simulink model "EMG_FES2(backup-18-05-2018)"  (R2014a)
settings: Solver=FixedStepDiscrete  StartTime=0.0  StopTime=inf  FixedStep=1/aFES.Fs  RelTol=1e-3
InitFcn:
  | mdl_initFcn_
StopFcn:
  | mdl_stopFcn_
values from neighbouring files (symbols this model uses):
  aFES = emgfes_feedback(aFES,[0,0,0,round(rand(1,2)*100)],1)    [emgfes_feedback_simulation.m]    (also in emgfesgui.m = a.aFES)
undefined symbols (not defined in the file or in its folder): analoginput, emgfes_feedback
libraries: dspmtrx3 x4, dspswit3 x3, simulink x2, ScienceStimHasomed_Lib x2, dspinverses x2, daqlib x1
settings Model: Creator=bethel.osuagwu  LastModifiedBy=bethel.osuagwu

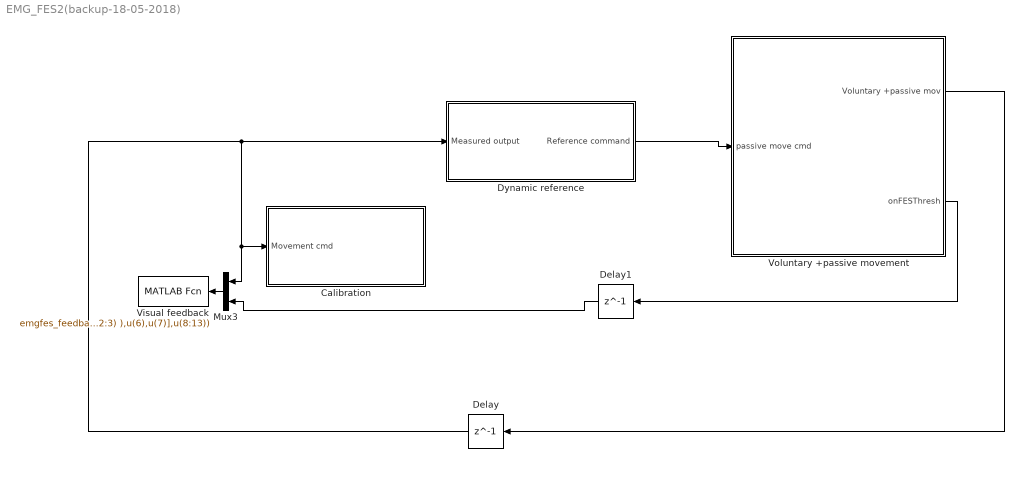
== system EMG_FES2(backup-18-05-2018) ==
  Calibration : Subsystem
  Delay : Delay  DelayLength=1  InitialCondition=zeros(7,1)
  Delay1 : Delay  DelayLength=1  InitialCondition=zeros(6,1)
  Dynamic reference : Subsystem
  Mux3 : Mux  Inputs=2
  Visual feedback : MATLABFcn  MATLABFcn=emgfes_feedback(aFES,[u(1), (u(2:3)'-aFES.activeSensorMin(2:3))./(aFES.activeSensorMax(2:3)-aFES.activeSensorMin(2:3) ),u(6),u(7)],u(8:13))  OutputDimensions=0
  Voluntary +passive movement : Subsystem
  wires:
  Dynamic reference/1(Reference command) -> Voluntary +passive movement/1(passive move cmd)
  Voluntary +passive movement/1(Voluntary +passive mov) -> Delay/1
  Delay/1 -> Dynamic reference/1(Measured output), Calibration/1(Movement cmd), Mux3/1
  Voluntary +passive movement/2(onFESThresh) -> Delay1/1
  Mux3/1 -> Visual feedback/1
  Delay1/1 -> Mux3/2

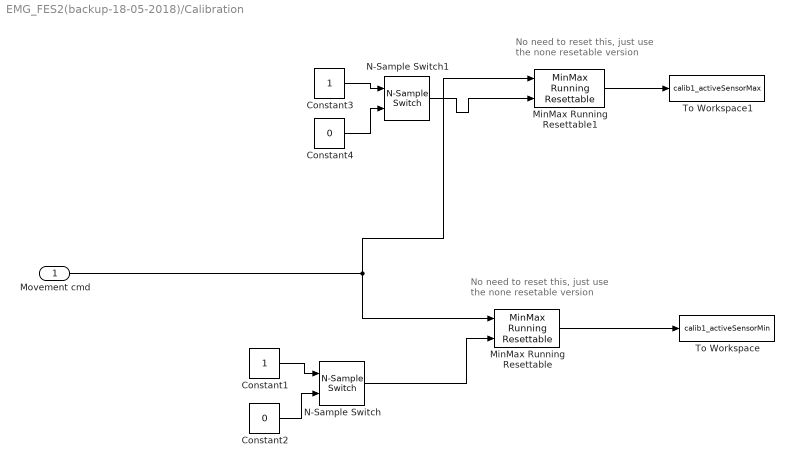
== system EMG_FES2(backup-18-05-2018)/Calibration ==
  note: No need to reset this, just use
      |  the none resetable version
  note: No need to reset this, just use
      |  the none resetable version
  Movement cmd : Inport
  Constant1 : Constant
  Constant2 : Constant  Value=0
  Constant3 : Constant
  Constant4 : Constant  Value=0
  MinMax Running Resettable : simulink/Math Operations/MinMax Running Resettable  Function=min  vinit=inf
  MinMax Running Resettable1 : simulink/Math Operations/MinMax Running Resettable  Function=max  vinit=-inf
  N-Sample Switch : dspswit3/N-Sample Switch  N=10000  reset=off  TriggerType=Rising edge  Ts=-1
  N-Sample Switch1 : dspswit3/N-Sample Switch  N=10000  reset=off  TriggerType=Rising edge  Ts=-1
  To Workspace : ToWorkspace  VariableName=calib1_activeSensorMin  SampleTime=-1
      settings: MaxDataPoints=1
  To Workspace1 : ToWorkspace  VariableName=calib1_activeSensorMax  SampleTime=-1
      settings: MaxDataPoints=1
  wires:
  N-Sample Switch1/1 -> MinMax Running Resettable1/2
  Constant1/1 -> N-Sample Switch/1
  MinMax Running Resettable1/1 -> To Workspace1/1
  MinMax Running Resettable/1 -> To Workspace/1
  N-Sample Switch/1 -> MinMax Running Resettable/2
  Constant2/1 -> N-Sample Switch/2
  Constant3/1 -> N-Sample Switch1/1
  Constant4/1 -> N-Sample Switch1/2
  Movement cmd/1 -> MinMax Running Resettable1/1, MinMax Running Resettable/1

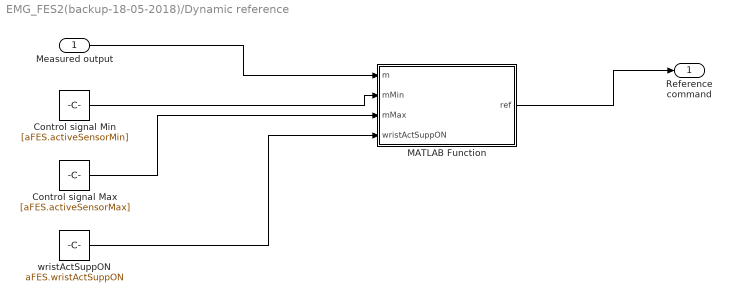
== system EMG_FES2(backup-18-05-2018)/Dynamic reference ==
  Measured output : Inport
  Control signal Max : Constant  Value=[aFES.activeSensorMax]
  Control signal Min : Constant  Value=[aFES.activeSensorMin]
  MATLAB Function : MATLAB Function  TreatAsAtomicUnit=on
  wristActSuppON : Constant  Value=aFES.wristActSuppON
  Reference command : Outport
  wires:
  Measured output/1 -> MATLAB Function/1(m)
  MATLAB Function/1(ref) -> Reference command/1
  Control signal Min/1 -> MATLAB Function/2(mMin)
  Control signal Max/1 -> MATLAB Function/3(mMax)
  wristActSuppON/1 -> MATLAB Function/4(wristActSuppON)

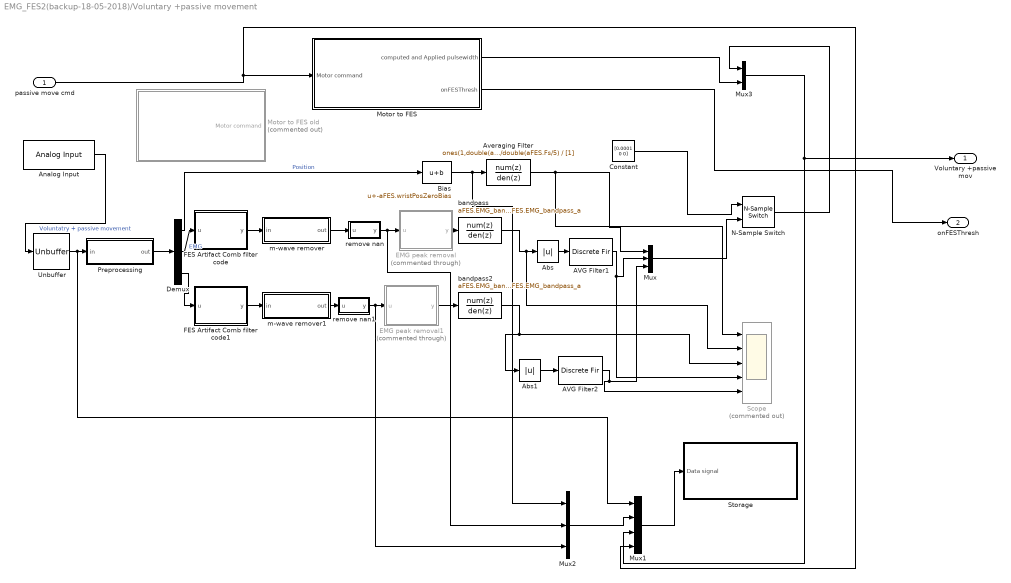
== system EMG_FES2(backup-18-05-2018)/Voluntary +passive movement ==
  passive move cmd : Inport
  " AVG Filter1" : DiscreteFir  Coefficients=ones(1,1000)/1000
  " AVG Filter2" : DiscreteFir  Coefficients=ones(1,1000)/1000
  Abs : Abs
  Abs1 : Abs
  Analog Input : daqlib/Analog Input  AcqMode=0  DeviceMenu=nidaq Dev1 (USB-6341 (BNC))  Device=nidaq Dev1 (USB-6341 (BNC))  ObjConstructor=analoginput('nidaq','Dev1')  SampleRate=1000  ActualRate=1000  SamplesPerFrame=2  InputType=Differential  NChannelsSelected=3  Channels=1$0$$2$#1$1$$2$#1$2$$2$#0$3$$1$#0$4$$1$#0$5$$1$#0$6$$1$#0$7$$1$#  NPorts=1 for all hardware channels  DataType=double
      settings: SignalType=Sample-based
  Averaging Filter : DiscreteFilter  Numerator=ones(1,double(aFES.Fs/5))/double(aFES.Fs/5)  Denominator=[1]
  Bias : Bias  Bias=-aFES.wristPosZeroBias
  Constant : Constant  Value=[0.0001 0 0]
  Demux : Demux  Outputs=3
  EMG peak removal : MATLAB Function  Commented=through  TreatAsAtomicUnit=on
  EMG peak removal1 : MATLAB Function  Commented=through  TreatAsAtomicUnit=on
  FES Artifact Comb filter code : MATLAB Function  TreatAsAtomicUnit=on
  FES Artifact Comb filter code1 : MATLAB Function  TreatAsAtomicUnit=on
  Motor to FES : Subsystem
  Motor to FES old : Subsystem  Commented=on
  Mux : Mux  Inputs=3
  Mux1 : Mux
  Mux2 : Mux  Inputs=3
  Mux3 : Mux  Inputs=2
  N-Sample Switch : dspswit3/N-Sample Switch  N=10  reset=off  TriggerType=Rising edge  Ts=-1
  Preprocessing : Subsystem
  Scope : Scope  Commented=on  NumInputPorts=5
      settings: YMin=-0.45~-0.15~-0.15~0~0  YMax=2.77556e-17~0.2~0.125~0.0125~0.015
  Storage : Subsystem
  Unbuffer : Unbuffer  SampleBasedProcessing=Same as frame based
  bandpass : DiscreteFilter  Numerator=aFES.EMG_bandpass_b  Denominator=aFES.EMG_bandpass_a
  bandpass2 : DiscreteFilter  Numerator=aFES.EMG_bandpass_b  Denominator=aFES.EMG_bandpass_a
  m-wave remover : Subsystem
  m-wave remover1 : Subsystem
  remove nan : MATLAB Function  TreatAsAtomicUnit=on
  remove nan1 : MATLAB Function  TreatAsAtomicUnit=on
  Voluntary +passive mov : Outport
  onFESThresh : Outport  Port=2
  wires:
  Analog Input/1 -> Unbuffer/1  "Voluntatry + passive movement"
  Demux/1 -> Bias/1  "Position"
  Abs/1 -> " AVG Filter1"/1
  " AVG Filter1"/1 -> Scope/4, Mux/2
  passive move cmd/1 -> Mux1/4, Motor to FES/1(Motor command)
  Demux/2 -> FES Artifact Comb filter code/1(u)  "EMG"
  Constant/1 -> N-Sample Switch/1
  N-Sample Switch/1 -> Mux3/1
  Unbuffer/1 -> Mux1/1, Preprocessing/1(in)
  Bias/1 -> Mux2/1, Averaging Filter/1
  Averaging Filter/1 -> Scope/1, Mux/1
  Abs1/1 -> " AVG Filter2"/1
  " AVG Filter2"/1 -> Scope/5, Mux/3
  Demux/3 -> FES Artifact Comb filter code1/1(u)
  FES Artifact Comb filter code/1(y) -> m-wave remover/1(in)
  EMG peak removal1/1(y) -> bandpass2/1
  Mux/1 -> N-Sample Switch/2
  Preprocessing/1(out) -> Demux/1
  m-wave remover/1(out) -> remove nan/1(u)
  FES Artifact Comb filter code1/1(y) -> m-wave remover1/1(in)
  EMG peak removal/1(y) -> bandpass/1
  bandpass/1 -> Scope/2, Abs/1
  bandpass2/1 -> Abs1/1, Scope/3
  remove nan/1(y) -> Mux2/2, EMG peak removal/1(u)
  remove nan1/1(y) -> Mux2/3, EMG peak removal1/1(u)
  m-wave remover1/1(out) -> remove nan1/1(u)
  Mux1/1 -> Storage/1(Data signal)
  Mux2/1 -> Mux1/2
  Motor to FES/1(computed and Applied pulsewidth) -> Mux3/2
  Motor to FES/2(onFESThresh) -> onFESThresh/1
  Mux3/1 -> Voluntary +passive mov/1, Mux1/3

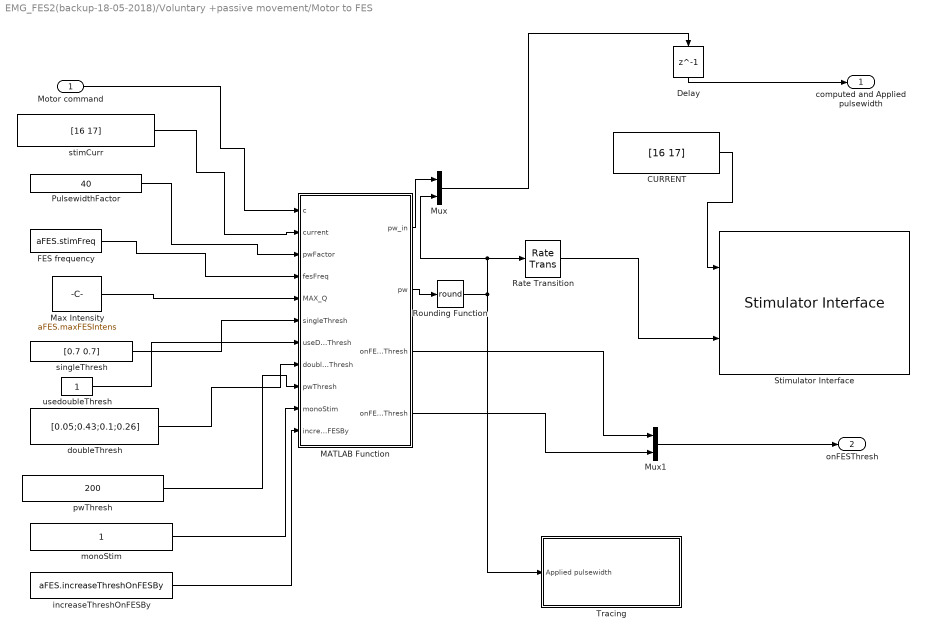
== system EMG_FES2(backup-18-05-2018)/Voluntary +passive movement/Motor to FES ==
  Motor command : Inport
  CURRENT : Constant  Value=[16 17]
  Delay : Delay  DelayLength=1  InitialCondition=0
  FES frequency : Constant  Value=aFES.stimFreq
  MATLAB Function : MATLAB Function  TreatAsAtomicUnit=on
  Max Intensity : Constant  Value=aFES.maxFESIntens
  Mux : Mux  Inputs=2
  Mux1 : Mux  Inputs=2
  PulsewidthFactor : Constant  Value=40
  Rate Transition : RateTransition
  Rounding Function : Rounding  Operator=round
  Stimulator Interface : ScienceStimHasomed_Lib/Stimulator Interface  Ts=33/aFES.Fs  com_port=COM9  channelstim=[1,2]  tsone=round((1/aFES.stimFreq)*1000)  tstwo=5  channellf=[]  nfactor=[]  outflag=off  dtflag=off
  Tracing : Subsystem
  doubleThresh : Constant  Value=[0.05;0.43;0.1;0.26]
  increaseThreshOnFESBy : Constant  Value=aFES.increaseThreshOnFESBy
  monoStim : Constant
  pwThresh : Constant  Value=200
  singleThresh : Constant  Value=[0.7 0.7]
  stimCurr : Constant  Value=[16 17]
  usedoubleThresh : Constant
  computed and Applied pulsewidth : Outport
  onFESThresh : Outport  Port=2
  wires:
  CURRENT/1 -> Stimulator Interface/1
  Motor command/1 -> MATLAB Function/1(c)
  MATLAB Function/2(pw) -> Rounding Function/1
  Rate Transition/1 -> Stimulator Interface/2
  stimCurr/1 -> MATLAB Function/2(current)
  Max Intensity/1 -> MATLAB Function/5(MAX_Q)
  doubleThresh/1 -> MATLAB Function/8(doubleThresh)
  MATLAB Function/1(pw_in) -> Mux/1
  Rounding Function/1 -> Tracing/1(Applied pulsewidth), Mux/2, Rate Transition/1
  pwThresh/1 -> MATLAB Function/9(pwThresh)
  FES frequency/1 -> MATLAB Function/4(fesFreq)
  PulsewidthFactor/1 -> MATLAB Function/3(pwFactor)
  monoStim/1 -> MATLAB Function/10(monoStim)
  Delay/1 -> computed and Applied pulsewidth/1
  usedoubleThresh/1 -> MATLAB Function/7(useDoubleThresh)
  singleThresh/1 -> MATLAB Function/6(singleThresh)
  Mux/1 -> Delay/1
  increaseThreshOnFESBy/1 -> MATLAB Function/11(increaseThreshOnFESBy)
  MATLAB Function/3(onFESSingleThresh) -> Mux1/1
  MATLAB Function/4(onFESDoubleThresh) -> Mux1/2
  Mux1/1 -> onFESThresh/1

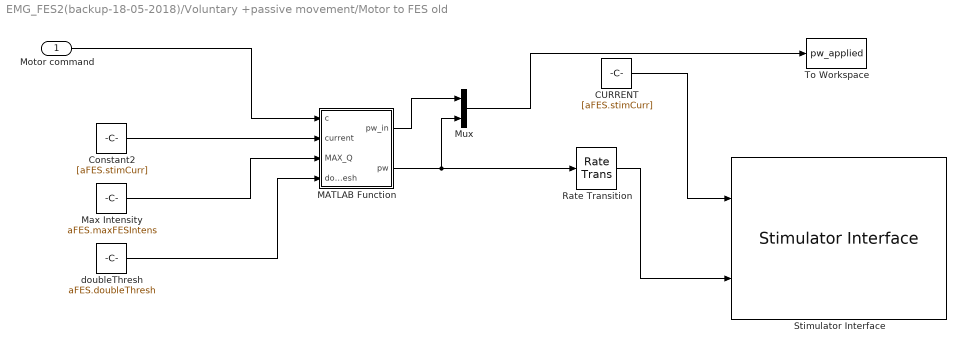
== system EMG_FES2(backup-18-05-2018)/Voluntary +passive movement/Motor to FES old ==
  Motor command : Inport
  CURRENT : Constant  Value=[aFES.stimCurr]
  Constant2 : Constant  Value=[aFES.stimCurr]
  MATLAB Function : MATLAB Function  TreatAsAtomicUnit=on
  Max Intensity : Constant  Value=aFES.maxFESIntens
  Mux : Mux  Inputs=2
  Rate Transition : RateTransition
  Stimulator Interface : ScienceStimHasomed_Lib/Stimulator Interface  Ts=33/aFES.Fs  com_port=COM9  channelstim=[1,2]  tsone=round((1/aFES.stimFreq)*1000)  tstwo=5  channellf=[]  nfactor=[]  outflag=off  dtflag=off
  To Workspace : ToWorkspace  VariableName=pw_applied  SampleTime=-1
  doubleThresh : Constant  Value=aFES.doubleThresh
  wires:
  Mux/1 -> To Workspace/1
  MATLAB Function/1(pw_in) -> Mux/1
  doubleThresh/1 -> MATLAB Function/4(doubleThresh)
  Max Intensity/1 -> MATLAB Function/3(MAX_Q)
  Constant2/1 -> MATLAB Function/2(current)
  Rate Transition/1 -> Stimulator Interface/2
  MATLAB Function/2(pw) -> Rate Transition/1, Mux/2
  Motor command/1 -> MATLAB Function/1(c)
  CURRENT/1 -> Stimulator Interface/1

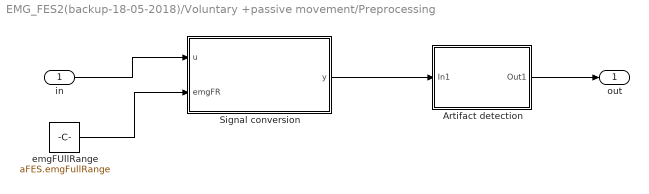
== system EMG_FES2(backup-18-05-2018)/Voluntary +passive movement/Preprocessing ==
  in : Inport
  Artifact detection : Subsystem
  Signal conversion : MATLAB Function  TreatAsAtomicUnit=on
  emgFUllRange : Constant  Value=aFES.emgFullRange
  out : Outport
  wires:
  Signal conversion/1(y) -> Artifact detection/1(In1)
  in/1 -> Signal conversion/1(u)
  Artifact detection/1(Out1) -> out/1
  emgFUllRange/1 -> Signal conversion/2(emgFR)

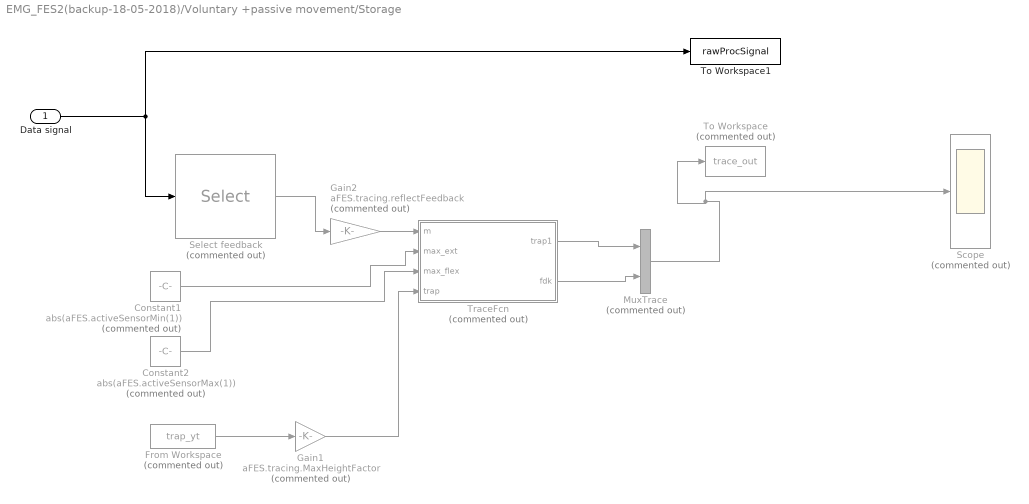
== system EMG_FES2(backup-18-05-2018)/Voluntary +passive movement/Storage ==
  Data signal : Inport
  Constant1 : Constant  Commented=on  Value=abs(aFES.activeSensorMin(1))
  Constant2 : Constant  Commented=on  Value=abs(aFES.activeSensorMax(1))
  From Workspace : FromWorkspace  Commented=on  VariableName=trap_yt  SampleTime=1/aFES.Fs  OutputAfterFinalValue=Setting to zero
  Gain1 : Gain  Commented=on  Gain=aFES.tracing.MaxHeightFactor
  Gain2 : Gain  Commented=on  Gain=aFES.tracing.reflectFeedback
  MuxTrace : Mux  Commented=on  Inputs=2
  Scope : Scope  Commented=on
      settings: TimeRange=100  YMin=-2.25  YMax=2  SaveName=ScopeData2
  Select feedback : Selector  Commented=on  InputPortWidth=9  Indices=[7]
  To Workspace : ToWorkspace  Commented=on  VariableName=trace_out  SampleTime=-1
  To Workspace1 : ToWorkspace  VariableName=rawProcSignal  SampleTime=-1
  TraceFcn : MATLAB Function  Commented=on  TreatAsAtomicUnit=on
  wires:
  TraceFcn/1(trap1) -> MuxTrace/1
  MuxTrace/1 -> Scope/1, To Workspace/1
  Gain1/1 -> TraceFcn/4(trap)
  Constant1/1 -> TraceFcn/2(max_ext)
  Constant2/1 -> TraceFcn/3(max_flex)
  Data signal/1 -> Select feedback/1, To Workspace1/1
  From Workspace/1 -> Gain1/1
  TraceFcn/2(fdk) -> MuxTrace/2
  Select feedback/1 -> Gain2/1
  Gain2/1 -> TraceFcn/1(m)

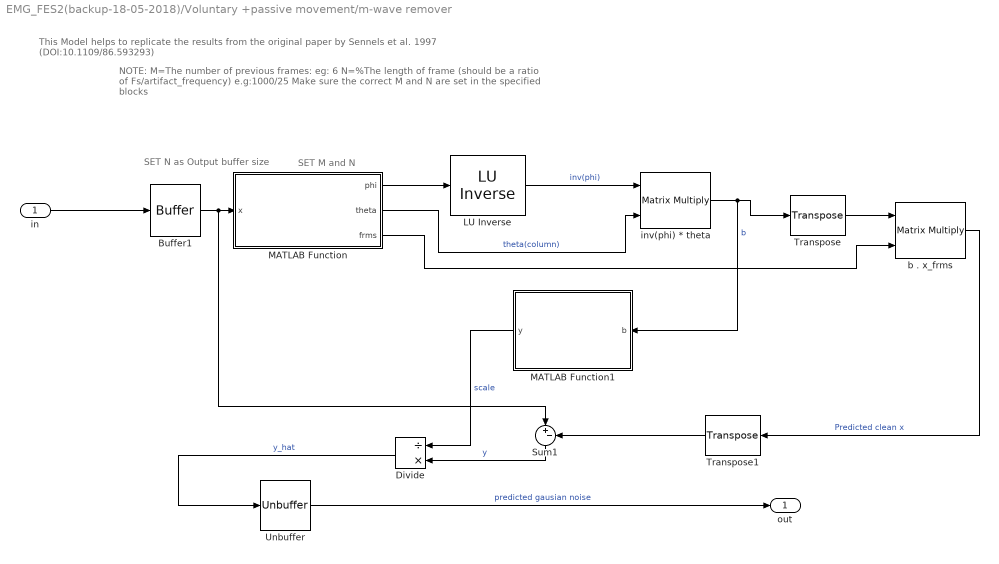
== system EMG_FES2(backup-18-05-2018)/Voluntary +passive movement/m-wave remover ==
  note: NOTE:
      | M=The number of previous frames: eg: 6
      | N=%The length of frame (should be a ratio of Fs/artifact_frequency) e.g:1000/25
      | Make sure the correct M and N are set in the specified blocks
  note: SET N as Output
      | buffer size
  note: SET M and N
  note: This Model helps to replicate the results from the original paper by Sennels et al. 1997 (DOI:10.1109/86.593293)
  in : Inport
  " LU Inverse" : dspinverses/ LU Inverse
  Buffer1 : Buffer  N=40  TreatMby1Signals=One channel
  Divide : Product  Inputs=/*
  MATLAB Function : MATLAB Function  TreatAsAtomicUnit=on
  MATLAB Function1 : MATLAB Function  TreatAsAtomicUnit=on
  Sum1 : Sum  Inputs=|+-
  Transpose : dspmtrx3/Transpose  Hermitian=off  overflowFlag=off
  Transpose1 : dspmtrx3/Transpose  Hermitian=off  overflowFlag=off
  Unbuffer : Unbuffer  SampleBasedProcessing=Same as frame based
  b . x_frms : Product  Multiplication=Matrix(*)
  inv(phi) * theta : Product  Multiplication=Matrix(*)
  out : Outport
  wires:
  Buffer1/1 -> Sum1/1, MATLAB Function/1(x)
  MATLAB Function/1(phi) -> " LU Inverse"/1
  MATLAB Function/2(theta) -> inv(phi) * theta/2  "theta(column)"
  " LU Inverse"/1 -> inv(phi) * theta/1  "inv(phi)"
  inv(phi) * theta/1 -> MATLAB Function1/1(b), Transpose/1  "b"
  Unbuffer/1 -> out/1  "predicted gausian noise"
  MATLAB Function/3(frms) -> b . x_frms/2
  Transpose/1 -> b . x_frms/1
  b . x_frms/1 -> Transpose1/1  "Predicted clean x"
  Transpose1/1 -> Sum1/2
  Sum1/1 -> Divide/2  "y"
  MATLAB Function1/1(y) -> Divide/1  "scale"
  Divide/1 -> Unbuffer/1  "y_hat"
  in/1 -> Buffer1/1

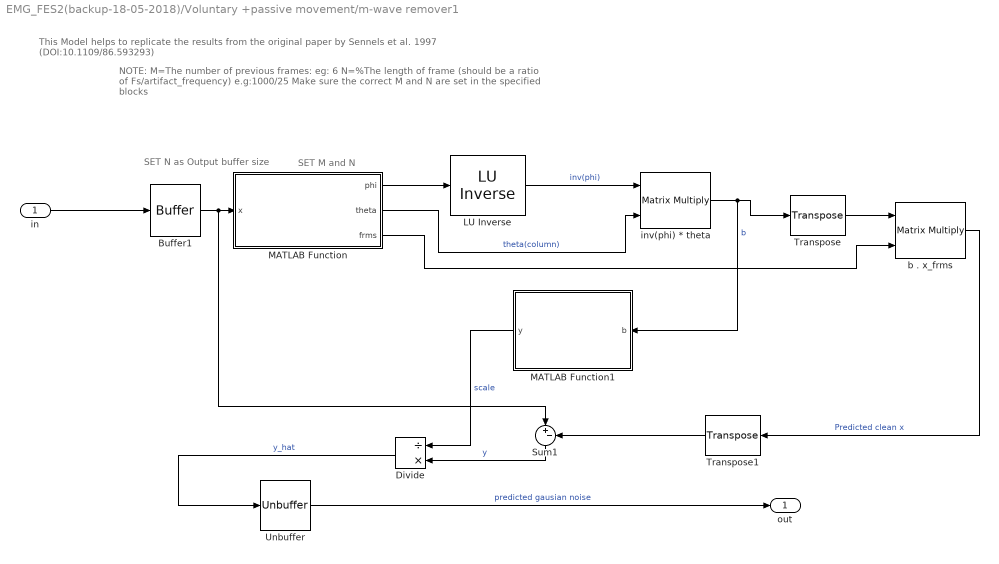
== system EMG_FES2(backup-18-05-2018)/Voluntary +passive movement/m-wave remover1 ==
  note: NOTE:
      | M=The number of previous frames: eg: 6
      | N=%The length of frame (should be a ratio of Fs/artifact_frequency) e.g:1000/25
      | Make sure the correct M and N are set in the specified blocks
  note: SET N as Output
      | buffer size
  note: SET M and N
  note: This Model helps to replicate the results from the original paper by Sennels et al. 1997 (DOI:10.1109/86.593293)
  in : Inport
  " LU Inverse" : dspinverses/ LU Inverse
  Buffer1 : Buffer  N=80  TreatMby1Signals=One channel
  Divide : Product  Inputs=/*
  MATLAB Function : MATLAB Function  TreatAsAtomicUnit=on
  MATLAB Function1 : MATLAB Function  TreatAsAtomicUnit=on
  Sum1 : Sum  Inputs=|+-
  Transpose : dspmtrx3/Transpose  Hermitian=off  overflowFlag=off
  Transpose1 : dspmtrx3/Transpose  Hermitian=off  overflowFlag=off
  Unbuffer : Unbuffer  SampleBasedProcessing=Same as frame based
  b . x_frms : Product  Multiplication=Matrix(*)
  inv(phi) * theta : Product  Multiplication=Matrix(*)
  out : Outport
  wires:
  Buffer1/1 -> Sum1/1, MATLAB Function/1(x)
  MATLAB Function/1(phi) -> " LU Inverse"/1
  MATLAB Function/2(theta) -> inv(phi) * theta/2  "theta(column)"
  " LU Inverse"/1 -> inv(phi) * theta/1  "inv(phi)"
  inv(phi) * theta/1 -> MATLAB Function1/1(b), Transpose/1  "b"
  Unbuffer/1 -> out/1  "predicted gausian noise"
  MATLAB Function/3(frms) -> b . x_frms/2
  Transpose/1 -> b . x_frms/1
  b . x_frms/1 -> Transpose1/1  "Predicted clean x"
  Transpose1/1 -> Sum1/2
  Sum1/1 -> Divide/2  "y"
  MATLAB Function1/1(y) -> Divide/1  "scale"
  Divide/1 -> Unbuffer/1  "y_hat"
  in/1 -> Buffer1/1

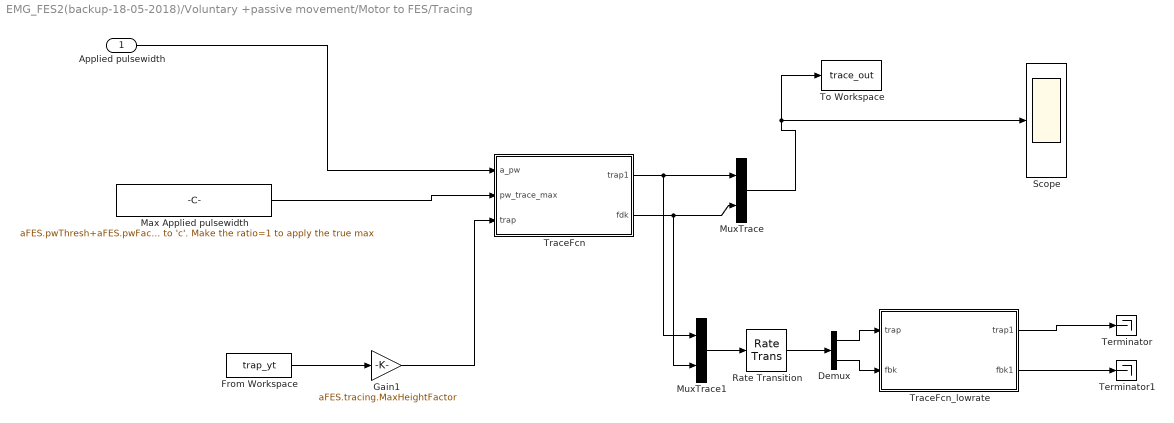
== system EMG_FES2(backup-18-05-2018)/Voluntary +passive movement/Motor to FES/Tracing ==
  Applied pulsewidth : Inport
  Demux : Demux  Outputs=2
  From Workspace : FromWorkspace  VariableName=trap_yt  SampleTime=1/aFES.Fs  OutputAfterFinalValue=Setting to zero
  Gain1 : Gain  Gain=aFES.tracing.MaxHeightFactor
  Max Applied pulsewidth : Constant  Value=aFES.pwThresh+aFES.pwFactor*[0.8,0.8] % so this multiplies pwFactor by a chosen ratio which is equivalent to 'c'. Make the ratio=1 to apply the true max
  MuxTrace : Mux  Inputs=2
  MuxTrace1 : Mux  Inputs=2
  Rate Transition : RateTransition  OutPortSampleTime=1/50
  Scope : Scope
      settings: TimeRange=100  YMin=-2.25  YMax=2  SaveName=ScopeData2
  Terminator : Terminator
  Terminator1 : Terminator
  To Workspace : ToWorkspace  VariableName=trace_out  SampleTime=-1
  TraceFcn : MATLAB Function  TreatAsAtomicUnit=on
  TraceFcn_lowrate : MATLAB Function  TreatAsAtomicUnit=on
  wires:
  TraceFcn/1(trap1) -> MuxTrace1/1, MuxTrace/1
  MuxTrace/1 -> To Workspace/1, Scope/1
  Gain1/1 -> TraceFcn/3(trap)
  Max Applied pulsewidth/1 -> TraceFcn/2(pw_trace_max)
  From Workspace/1 -> Gain1/1
  TraceFcn/2(fdk) -> MuxTrace/2, MuxTrace1/2
  Applied pulsewidth/1 -> TraceFcn/1(a_pw)
  TraceFcn_lowrate/1(trap1) -> Terminator/1
  TraceFcn_lowrate/2(fbk1) -> Terminator1/1
  MuxTrace1/1 -> Rate Transition/1
  Rate Transition/1 -> Demux/1
  Demux/1 -> TraceFcn_lowrate/1(trap)
  Demux/2 -> TraceFcn_lowrate/2(fbk)

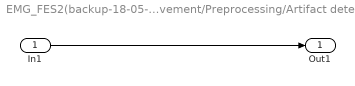
== system EMG_FES2(backup-18-05-2018)/Voluntary +passive movement/Preprocessing/Artifact detection ==
  In1 : Inport
  Out1 : Outport
  wires:
  In1/1 -> Out1/1

== matlab function EMG_FES2(backup-18-05-2018)/Dynamic reference/MATLAB Function ==
  data: m input; mMin input; ref output; mMax input; wristActSuppON input
function ref   = fcn(m,mMin,mMax,wristActSuppON)
%#codegen
%m(1)=position/force, extension should have negative values while flexion
%have positiove values and 0 is neutral
%m(2:3) measure of ext. EMG and Flex EMG power respectively (i.e.
%m(3)->extension and m(3)->flexion
%
%mMin and mMax are the calibration min and max resp. for m values
%
%
%
%SeSsions maked as modules can be removed without causing too much harm to
%the system, removing them just removes their minor function which does not
%affect the main system
%
%
persistent t_blocking ref_mem act_chnl_mem act_mem;
% act_chnl_mem ={0:3}. Tells us which 'vitual' channel is on. 0:none;
% 1:extension; 2:flexion; 3:tenodesis grip; 4:tenodesis release; 5:both
% flexion and extension

%assert(m<=3);

ref=[0,0];

%% General parameters 

%These should be determin at the starte of every test and should be input to the fucntion
mMaxVolPercent=[1;0.9999999;0.999999];%The percentage of max voluntary value to be used as the actuall Max. E.g 0.5, means  50% of mMax is used as the actual mMax while a value of 1 means to use full mMax as mMax
mMax_=mMax.*mMaxVolPercent;%Rescale mMax

wristMax=mMax_(1);
wristMin=mMin(1);

pFlexRefMax=mMax_(3);
pFlexRefMin=mMin(3);

pExtRefMax=mMax_(2);
pExtRefMin=mMin(2);

tenodesisON=[0;0];%1=allow tenodesis; 0=No tenodesis: tenodesisON(1) for tenodesis grip. tenodesisON(2) for tenodesis release

wristExtTenoPerc =0.95;% The percentage of max wrist extension at which forced(i.e based only on wrist) tenodesis grip should be activated
wristFlexTenoPerc =0.97;%The percentage of max wrist flexion at which forced (i.e based only on wrist) tenodesis release should be activated

extTenoPerc =0.80;% The percentage of max wrist extension at which activated(i.e based on both finger and wrist, Tenodesis proper) tenodesis grip should be activated
flexTenoPerc =0.80;%The percentage of max wrist flexion at which activated (i.e based on both finger and wrist Tenodesis proper) tenodesis release should be activated

act_opposeLowerPerc=0.7;%{1= no lowering of activation threshold, 0=lower activation threshold to zero}the percentage to lower the activation of an opposing movement to give it a chance to activate

%calculate the activation threshold as a set percentage above the the
%minimun signal
act_thresh_ext=mMin(2)+0.05*mMin(2);
act_thresh_flex=mMin(3)+0.05*mMin(3);

%%Add small activation based on goniometer position. BUT FOR BETTER CONTROL, TURN THIS OFF IF
%%FES INTENSITY IS HIGH TO PRODUCE LARGE MOVEMENT \KODE*~#1.
%wristActSuppON=[1;1];%{see \KODE *~#1)true to turn ON supplimentary activation when the wrist is moved above threshold:: wristActSuppON(1)=>ext; wristActSuppON(2)=>flex
wristActThresh =[wristMin;wristMax]*0.05; %the activation threshold for wrist movement

%Blocking window
oppositeRefracWin =1000;%The number of samples for which to refrain from imidiate opposite movement



%% Begin
if(isempty(t_blocking))    
   ref=[m(2),m(3)];%Make the current reference
   ref_mem=ref;
   t_blocking=0;
   act_chnl_mem=0;
   act_mem=0;
   return;
end

%update blocking timing
if t_blocking 
    if t_blocking>=oppositeRefracWin %refractory period of samples
        t_blocking=0;
    else
        t_blocking=t_blocking+1;
    end
end


%% Compute relative power
m(3)=(m(3)-pFlexRefMin)/(pFlexRefMax-pFlexRefMin);
m(2)=(m(2)-pExtRefMin)/(pExtRefMax-pExtRefMin);



%% Compute channel selection parameters
wristFlex=0;
wristExt=0;
tenoGras=0;
tenoRelease=0;
wristActSupp=[0;0];% 
if m(1)>0 
    wristFlex=1;%flex
    act_thresh_ext=act_thresh_ext*act_opposeLowerPerc;% lower the activation threshold of extension when the wrist is flex( Note that this might have been done by an external block):
    
    %%wrist position adds a bit of activation for flexion
    if m(1)>wristActThresh(2) && wristActSuppON(2)
        wristActSupp(2)=m(3)*0.3;
    end
    
    if(tenodesisON(2))
        if m(1)>wristMax*wristFlexTenoPerc 
            tenoRelease=1;   
        end
    end
    
else
    wristExt=1;%extension
    act_thresh_flex=act_thresh_flex*act_opposeLowerPerc ;% lower the activation threshold of flexion when the wrist extended: (Note that this might have been done by an external block)
    
    %%wrist position adds a bit of activation for extension
    if m(1)<wristActThresh(1) && wristActSuppON(1)
        wristActSupp(1)=m(2)*0.3;
    end
    
    if m(1)<wristMin*wristExtTenoPerc %TODO: check ik if (tenodesisON(1)==1
        tenoGras=1;
    end
 
end

%% Are current values greater than their thresh hold
pFlex=0;
if m(3)>act_thresh_flex
    pFlex=1;
end

pExt=0;
if m(2)>act_thresh_ext
    pExt=1;
end


%% Classify flexion and extension
isFlex=double(m(2)<m(3));

isExt=1-isFlex;
if(wristExt && pFlex)
    %So the wrist is extended but the fingers are closing
    isFlex=1; %reinforce that flexion should be on
end
if(wristFlex && pExt)
    %so the writs is flexed but the fingers are opening
    isExt=1;%reinforce that extension should be on
end

%Total flexion
isFlex=isFlex+pFlex+wristFlex;
%Total extension
isExt=isExt+pExt+wristExt;

 
%% Tenodesis proper (fingers and wrists)
if (wristFlex && m(1)>wristMax*flexTenoPerc && 1.5*m(2)>m(3)) && tenodesisON(2)
    %This is another way to turn on tenodesis release
    tenoRelease=tenoRelease+1;
end

if(wristExt && m(1)<wristMin*extTenoPerc && 1.5*m(3)>m(2)) && tenodesisON(1)
    %This is another way to turn on tenodesis grip
    tenoGras=tenoGras+1;
end


%% Compute ref
if tenoGras && tenodesisON(1)%i.e Tenodesis grip
    ref=[m(2),m(3)];% +wristActSupp;
    ref(2)=ref(2) + ref(2)*tenoGras*0.5; %cheat for flexion by the magnitude of the tenoGras
    act_chnl=3; %See header for the meaning of activated channels
elseif tenoRelease && tenodesisON(2)%i.e Tenodesis release
    ref=[m(2),m(3)];%+wristActSupp;
    ref(1)=ref(1) + ref(1)*tenoRelease*0.5; %cheat for flexion by the magnitude of the tenoRelease
    act_chnl=4; %See header for the meaning of activated channels
elseif isFlex>isExt
    ref=[0,m(3)];
    ref(2)=ref(2)+wristActSupp(2);
    act_chnl=2;
elseif isExt>isFlex
    ref=[m(2),0];
    ref(1)=ref(1)+wristActSupp(1);
    act_chnl=1;
elseif isExt && isFlex && isExt==isFlex
    ref=[m(2),m(3)];%+wristActSupp;
    act_chnl=5;
else   
    ref=[0,0];
    act_chnl=0;
end
act=sum(ref);   

%% Check if we can block activation
%%implements blocking of immediate opposite movement
if ~t_blocking || act_chnl==act_chnl_mem && act>act_mem% The operator precidence here should lead to the correct operation
    t_blocking=1;% start blocking of further imidiate opposite change
else
    ref=ref_mem; 
end


%% Save to mem
if(ref(1)~=ref_mem(1) || ref(2)~=ref_mem(2))
    act_mem=act;
    act_chnl_mem=act_chnl;
    ref_mem=ref;
    
end

== matlab function EMG_FES2(backup-18-05-2018)/Voluntary +passive movement/FES Artifact Comb filter code ==
  data: u input; y output
function y  = fcn(u)
%#codegen

persistent u_mem;
fes_freq=25;%FES frequency
Fs=1000;%EMG/data samplerate
K=40;%round(Fs/fes_freq); %Comb filter order = (1/fes_freq)*Fs
a=-1;%{-1 to 0}
if isempty(u_mem)
    u_mem=zeros(K,1);
end





%% Comb filtering
% Forward comb
y=u+ a*u_mem(1);



u_mem(1:end-1)=u_mem(2:end);
u_mem(end)=u;



end





%

== matlab function EMG_FES2(backup-18-05-2018)/Voluntary +passive movement/Motor to FES/MATLAB Function ==
  data: pw_in output; c input; current input; pw output; pwFactor input; fesFreq input; MAX_Q input; singleThresh input; useDoubleThresh input; doubleThresh input; pwThresh input; monoStim input; increaseThreshOnFESBy input; onFESSingleThresh output; onFESDoubleThresh output
function [pw_in,pw,onFESSingleThresh,onFESDoubleThresh] = fcn(c,current,pwFactor,fesFreq,MAX_Q,singleThresh,useDoubleThresh,doubleThresh,pwThresh,monoStim,increaseThreshOnFESBy)
%#codegen
% c: is the controller output. Normally expressed as percentage activation
% above basseline and normalised with the Max ativation.
% current: is a vector(1 ele/chnl) of FES current in milliamps
% pwFactor: is the factor used to convert activation to pulsewidth 
% fesFreq: is the FES frequency
% MAX_Q:= eg.5000;%maxmum FES intensity =current x pulsewidth *freq
% useDoubleThresh: %When this variable evaluates to true, doubleThresh is applied
% doubleThresh: {[OFF thresh ch1; ON thresh ch1];[OFF thresh ch2; ON thresh ch2]}is the double thresh similer to that by Ambrosini
% pwThresh: is the starting pulsewidth once activation reaches
%threshold
% monoStim:(also see run_afes.m) {0<=monoStim<=1} When 1=> only one channel is allowed to be
% active at a time; when 0=>the two channels are allowed to be active
% simutanousely etc;  The pulsewidth of the channel other than the A MAIN
% active channel is scaled by S(1-monoStim) to a percentage of its
% activity. 
% increaseThreshOnFESBy: When true the threshold will be increased by this amount during stimulation, making it harder to activate and easier to deactivate
%
% pw_in: Exact computed pulsewidth
% pw: The actual pulsewidth that will be applied,
% onFESSingleThresh: The single threshold used when FES is ON
% onFESDoublThresh: Double thresh used when FES is ON
%
% NOTE: Any section of the code labelled 'Module' is independent and
% therefore can be removed without affecting other functions 
persistent   FES_ON pw_smooth MAIN_FES_ON c_mem;


if isempty(pw_smooth)
    %c_mem=zeros(30,2);
    FES_ON=[0;0];
    pw_smooth=[0;0];
    [~,MAIN_FES_ON]=max(c);% {1:noOfChannels} MAIN_FES_ON is considered the main active channel even when both channels are active. The current MAIN_FES_ON channel must become inactive when the other channel becomes active
    c_mem=[0,0];
end

onFESSingleThresh=singleThresh;
onFESDoubleThresh=doubleThresh;

%FES_ON_prev=FES_ON;

%% (Module) Avoid spikes in Stimulation
% if false
% c(dcdt>0.5)=median(c_mem);
% %upadte memory of controller output
%  c_mem(1:end-1,:)=c_mem(2:end,:);
%  c_mem(end,:)=c;
% end
%% (Module) Increase the threshold when stimulation is on
if(any(increaseThreshOnFESBy))
    if (any(FES_ON) && max(c_mem)>=0.8 ) % i.e if any channel is ON and it is significantly active
        if(useDoubleThresh)
            %We increase the threshold by the set percentage making sure it is still below 100%
            if(increaseThreshOnFESBy(1))
                % First for channel 1
                doubleThresh(1)=min([doubleThresh(1)+increaseThreshOnFESBy(1),0.90]);
                doubleThresh(2)=min([doubleThresh(2)+increaseThreshOnFESBy(1),0.95]);
                if(doubleThresh(1)>doubleThresh(2))
                    doubleThresh(2)=0.95;
                end
            end
            if(increaseThreshOnFESBy(2))
                % Then for channel 2
                doubleThresh(3)=min([doubleThresh(3)+increaseThreshOnFESBy(2),0.90]);
                doubleThresh(4)=min([doubleThresh(4)+increaseThreshOnFESBy(2),0.95]);
                if(doubleThresh(3)>doubleThresh(4))
                    doubleThresh(4)=0.95;
                end
            end
            
            onFESDoubleThresh=doubleThresh;
        else
            %We increase the threshold by the set percentage making sure it is still below 100%
            if(increaseThreshOnFESBy(1))
                singleThresh(1)=min([singleThresh(1)+increaseThreshOnFESBy(1),0.95]);
            end
            if(increaseThreshOnFESBy(2))
                singleThresh(2)=min([singleThresh(2)+increaseThreshOnFESBy(2),0.95]);
            end
            
            onFESSingleThresh=singleThresh;
        end
    end
   
    
end


%% (Module) Limit value of 'c'
c_max=20.5; % Max value allowed for 'c'
for nc=1:2
    if(c(nc)>c_max)
        c(nc)=c_mem(nc);
        'Block - Motor to FES: Setting channel to prev val b/c overactivation on Channel: '
        nc
    end
end
%c_mem=c;




%% compute pulsewidth
% Implement double threshold 
if(useDoubleThresh)%% so currently useDoubleThresh cannot be se separatly each channel
    pw=[0;0];
    for chni=1:2
        if FES_ON(chni) %If the channel is ON, check if it has dropped below first double thresh
            if c(chni)<doubleThresh(1+2*(chni-1))%If the channel has dropped below the first thresh, then turn it OFF
                pw(chni)=0;
                FES_ON(chni)=0;
            else %But if the channel is still above the OFF thresh, then proportionally set the pw
                %pw(chni)=200+c(chni)*30;%
                pw(chni)=pwThresh+c(chni)*pwFactor;
                FES_ON(chni)=1;
            end
        else %But is the channel currently OFF, Check if it has activation above ON thresh
            if c(chni)>doubleThresh(2+2*(chni-1))% If the activation is above ON thresh,then proportionally set the pw
                %pw(chni)=200+c(chni)*30;%
                pw(chni)=pwThresh+c(chni)*pwFactor;
                FES_ON(chni)=1;
            else %but if it is still under the ON thresh, make sure that it is set to off
                pw(chni)=0;
                FES_ON(chni)=0;
            end
        end
    end
    
else %Double threshold is disabled, need to use singleThresh
    pw=[0;0];
    for chni=1:2
        if c(chni)>singleThresh(chni)
            pw(chni)=pwThresh+c(chni)*pwFactor;
            FES_ON(chni)=1;
        else
            pw(chni)=0;
            FES_ON(chni)=0;
        end
    end
    %pw=(c).*pwFactor;%OR %pw=pwThresh+(c).*pwFactor;
      
    %pw(pw<0)=0;
    %pw(pw>50)=pw(pw>50)+10;%add a bias
    %pw(pw<50)=0;
    %pw=pw*5;
    %FES_ON=double(pw>0);
    
end



%% (Module) Stimulate only one channel at a time
%%%%THIS MAY NOT BE WORKING PROPERLY

if monoStim && all(FES_ON)%Has both channel been set to active?
    % Determin the main active Channel
%     if ~FES_ON(MAIN_FES_ON)==1;
%       if FES_ON(3-MAIN_FES_ON)==1;
%           MAIN_FES_ON=3-MAIN_FES_ON;
%       end
%     end    
    pw(3-MAIN_FES_ON)=pw(3-MAIN_FES_ON)*(1-monoStim);%Select the channel that was OFF and set it to remain OFF(i.e x (1-mnonStim)=0) or reduce its activation according to '1-monoStim'
    
%////////////////////////////////////////////////////////////////////
%     if ~(numel(pw(~FES_ON_prev))==2)
%         
%         pw(~FES_ON_prev)=pw(~FES_ON_prev)*(1-monoStim);%Select the channel that was previously OFF and leave it on or reduce its activation according to 'monoStim'
%         if(monoStim==1)
%             FES_ON=FES_ON_prev;
%         end
%     end
%////////////////////////////////////////////////////////////////////
elseif any(FES_ON)
    [~,MAIN_FES_ON]=max(FES_ON);
else
    %you can favour a particular channel here eg: MAIN_FES_ON=2; or just do
    %nothing to leave the the prevously active chnnel
end




%% Limit max Intensity of FES ::NOTE:  OPEN THIS TO APPLY LIMITATIONS
% q=current.*pw*fesFreq;
% q_=q>MAX_Q;
% for nq=1:length(q_)
%     if q_(nq)
%         pw(nq)=MAX_Q/(current(nq)*fesFreq);
%         'Motor to FES: limits [ch,pulsewidth_limit]'
%         [nq pw(nq)]
%     end
% end



%% The estimated pw is essentially our input pw
pw_in=pw;% If no further modification below, then pw_in==pw


%% (Module)Controller output based change in stimulation for opposing movement assistance



%% (Module)Error based change in stimulation for opposing movement assistance


%% (Module) Smoothness controller for pw
pw_step=0.1;%(TODO: should be a function of max pw and samplerate)allowed positive step chnage per sample
pw=abs(pw_smooth+sign(pw-pw_smooth)*pw_step); %the abs here is fine as far as the step size is small(e.g <5)
%pw(pw<pw_step)=0;NOTE open this 
pw_smooth=pw;
%-----------------------------

%% Update memory
c_mem=c; % update c incase any part of the part of the script needs it.

== matlab function EMG_FES2(backup-18-05-2018)/Voluntary +passive movement/m-wave remover/MATLAB Function ==
  data: x input; phi output double; theta output; frms output
function [phi,theta,frms] = fcn(x)
%#codegen
persistent t_sample phi_mem  frms_mem ;

%General param
M=6; %The number of previous frames 
N=40; %The length of frame (should be a ratio of Fs/artifact_frequency)

% Performance parameter
freshPhi =1;% when =1:recompute phi(covariance matix) all the phi; when =0:update phi with only new values

if isempty(t_sample)
    t_sample=0;
    frms_mem=zeros(M,N);
    
    phi_mem=zeros(M,M);
end
t_sample=t_sample+1;

%make x a row vector
x=x';


%% compute phi
frms=frms_mem;
%equ 7 and 8
if(freshPhi)
    % compute phi fresh all the time
    phi=(frms*frms');
else
    %we can compute only the required column (first) and row (first)of phi
    %matrix and push the new values into phi
    phi_mem(2:end,2:end)=phi_mem(1:end-1,1:end-1);
    phi_mem(1,:)=frms(1,:)*frms';
    phi_mem(:,1)=phi_mem(1,:)';
    %phi-phi_mem
    phi=phi_mem;
end


%% compute theta
theta=(x*frms')';
%t_sample
%if t_sample==15
%    y=4;
%end


%% update frame
frms_mem(2:end,:)=frms_mem(1:end-1,:);
frms_mem(1,:)=x;

== matlab function EMG_FES2(backup-18-05-2018)/Voluntary +passive movement/FES Artifact Comb filter code1 ==
  data: u input; y output
function y  = fcn(u)
%#codegen

persistent u_mem;
fes_freq=25;%FES frequency
Fs=1000;%EMG/data samplerate
K=40;%round(Fs/fes_freq); %Comb filter order = (1/fes_freq)*Fs
a=-1;%{-1 to 0}
if isempty(u_mem)
    u_mem=zeros(K,1);
end





%% Comb filtering
% Forward comb
y=u+ a*u_mem(1);



u_mem(1:end-1)=u_mem(2:end);
u_mem(end)=u;
end





%

== matlab function EMG_FES2(backup-18-05-2018)/Voluntary +passive movement/EMG peak removal1 ==
  data: u input; y output
function y  = fcn(u)
%#codegen
%peak removal
peak_thresh=0.5;
dmdt_thresh=0.3;
blocking_win=50;
persistent u_mem t_;
if isempty(u_mem)
    u_mem=zeros(1000,1);
    t_=0;
end

if (dmdt_thresh<abs(u)-abs(u_mem(end))&& t_==0)%if the change in value to too large  then block with no stats
    t_=1;
else   
    if((abs(u)>peak_thresh || dmdt_thresh<abs(u)-abs(u_mem(end))) && t_==0) %detect high amplitude,peak, and start blocking
        if(abs(u)>std(u_mem))
            t_=1;
        end
    end

    
end


if t_
    u=0;%block
   t_=t_+1;
end
if(t_==blocking_win) %stop blocking after n samples
    t_=0; 
end

u_mem(1:end-1)=u_mem(2:end);
u_mem(end)=u;
y=u;
end





%

== matlab function EMG_FES2(backup-18-05-2018)/Voluntary +passive movement/EMG peak removal ==
  data: u input; y output
function y  = fcn(u)
%#codegen
%peak removal
peak_thresh=0.5;
dmdt_thresh=0.3;
blocking_win=50;
persistent u_mem t_;
if isempty(u_mem)
    u_mem=zeros(1000,1);
    t_=0;
end

if (dmdt_thresh<abs(u)-abs(u_mem(end))&& t_==0)%if the change in value to too large  then block with no stats
    t_=1;
else   
    if((abs(u)>peak_thresh || dmdt_thresh<abs(u)-abs(u_mem(end))) && t_==0) %detect high amplitude,peak, and start blocking
        if(abs(u)>std(u_mem))
            t_=1;
        end
    end

    
end


if t_
    u=0;%block
   t_=t_+1;
end
if(t_==blocking_win) %stop blocking after n samples
    t_=0; 
end

u_mem(1:end-1)=u_mem(2:end);
u_mem(end)=u;
y=u;
end





%

== matlab function EMG_FES2(backup-18-05-2018)/Voluntary +passive movement/remove nan ==
  data: u input; y output
function y  = fcn(u)
%#codegen

y=u;
if isnan(y)
    y=0;
end





%

== matlab function EMG_FES2(backup-18-05-2018)/Voluntary +passive movement/remove nan1 ==
  data: u input; y output
function y  = fcn(u)
%#codegen

y=u;
if isnan(y)
    y=0;
end





%

== matlab function EMG_FES2(backup-18-05-2018)/Voluntary +passive movement/m-wave remover/MATLAB Function1 ==
  data: b input; y output
function y = fcn(b)
%#codegen


y = sqrt(1+sum(b.^2));
%       OR
%y = (1+sum(b));%approximated for speed

== matlab function EMG_FES2(backup-18-05-2018)/Voluntary +passive movement/m-wave remover1/MATLAB Function ==
  data: x input; phi output double; theta output; frms output
function [phi,theta,frms] = fcn(x)
%#codegen
persistent t_sample phi_mem  frms_mem ;

%General param
M=6; %The number of previous frames 
N=80; %The length of frame (should be a ratio of Fs/artifact_frequency)

% Performance parameter
freshPhi =1;% when =1:recompute phi(covariance matix) all the phi; when =0:update phi with only new values

if isempty(t_sample)
    t_sample=0;
    frms_mem=zeros(M,N);
    
    phi_mem=zeros(M,M);
end
t_sample=t_sample+1;

%make x a row vector
x=x';


%% compute phi
frms=frms_mem;
%equ 7 and 8
if(freshPhi)
    % compute phi fresh all the time
    phi=(frms*frms');
else
    %we can compute only the required column (first) and row (first)of phi
    %matrix and push the new values into phi
    phi_mem(2:end,2:end)=phi_mem(1:end-1,1:end-1);
    phi_mem(1,:)=frms(1,:)*frms';
    phi_mem(:,1)=phi_mem(1,:)';
    %phi-phi_mem
    phi=phi_mem;
end


%% compute theta
theta=(x*frms')';
%t_sample
%if t_sample==15
%    y=4;
%end


%% update frame
frms_mem(2:end,:)=frms_mem(1:end-1,:);
frms_mem(1,:)=x;

== matlab function EMG_FES2(backup-18-05-2018)/Voluntary +passive movement/m-wave remover1/MATLAB Function1 ==
  data: b input; y output
function y = fcn(b)
%#codegen


y = sqrt(1+sum(b.^2));
%       OR
%y = (1+sum(b));%approximated for speed

== matlab function EMG_FES2(backup-18-05-2018)/Voluntary +passive movement/Storage/TraceFcn ==
  data: m input; max_ext input; max_flex input; trap input; trap1 output; fdk output
function [trap1,fdk]    = fcn(m,max_ext,max_flex,trap)
%#codegen
%coder.extrinsic('plot','hold');
% persistent ts;
% if isempty(ts)
%     ts=0;
%     %m_mem=zeros(10*1000,1);
% end
%m_mem(1:end-1)=m_mem(2:end);
%m_mem(end)=m(1);

%scale extension
if(m(1)>0)
    m(1)=m(1)/max_ext;
elseif m(1)<0
    m(1)=m(1)/max_flex;
end
    
%ts=ts+1;
 trap1=trap;
 
 fdk=m(1);
 
%stopSingnal=0;
%  if(ts==length(trap))
%      stopSingnal=1;
%  end

== matlab function EMG_FES2(backup-18-05-2018)/Voluntary +passive movement/Motor to FES old/MATLAB Function ==
  data: pw_in output; c input; current input; pw output; MAX_Q input; doubleThresh input
function [pw_in,pw] = fcn(c,current,MAX_Q,doubleThresh)
%#codegen
% c is the controller output
% dcdt is the derivative of c
%MAX_Q= eg.5000;%maxmum intensity =current x pulsewidth
persistent  FES_ON pw_smooth;

pMax=300;
if isempty(pw_smooth)
    %c_mem=zeros(30,2);
    FES_ON=[0;0];
    pw_smooth=[0;0];
end


%% (Module) Avoid spikes in Stimulation
% if false
% c(dcdt>0.5)=median(c_mem);
% %upadte memory of controller output
%  c_mem(1:end-1,:)=c_mem(2:end,:);
%  c_mem(end,:)=c;
% end

%compute pulsewidth
if(doubleThresh(2))
    pw=[0;0];
    for chni=1:2
        if FES_ON(chni)
            if c(chni)<doubleThresh(1)
                pw(chni)=0;
                FES_ON(chni)=0;
            else
                pw(chni)=200+c(chni).*30;
                FES_ON(chni)=1;
            end
        else %it is currently off
            if c(chni)>doubleThresh(2)
                pw(chni)=200+c(chni).*30;
                FES_ON(chni)=1;
            else
                pw(chni)=0;
                FES_ON(chni)=0;
            end
        end
    end
    
else
    pw=(c).*pMax;
    pw(pw<0)=0;
    %pw(pw>50)=pw(pw>50)+10;%add a bias
    pw(pw<50)=0;
end

%% Limit max Intensity of FES
q=current.*pw;
q_=q>MAX_Q;
for nq=1:length(q_)
    if q_(nq)
        pw(nq)=MAX_Q/current(nq);
        'Motor to FES: limits [ch,pulsewidth_limit]'
        [nq pw(nq)]
    end
end

%% The estimated pw is essentially our input pw
pw_in=pw;% If no further modification below, then pw_in==pw


%% (Module)Controller output based change in stimulation for opposing movement assistance



%% (Module)Error based change in stimulation for opposing movement assistance


%% (Module) Smoothness controller for pw
pw_step=0.2;%(TODO: should be a function of max pw and samplerate)allowed positive step chnage per sample
pw=abs(pw_smooth+sign(pw-pw_smooth)*pw_step); %the abs here is fine as far as the step size is small(e.g <5)
%pw(pw<pw_step)=0;NOTE open this 
pw_smooth=pw;
%-----------------------------

== matlab function EMG_FES2(backup-18-05-2018)/Voluntary +passive movement/Motor to FES/Tracing/TraceFcn ==
  data: a_pw input; pw_trace_max input; trap input; trap1 output; fdk output
function [trap1,fdk]    = fcn(a_pw,pw_trace_max,trap)
%#codegen
% a_pw: The current applied pulsewith
% pw_trace_max: used the value corresponding to 1 on the tracing window
% trap: The current sample of trapezium
%
%coder.extrinsic('plot','hold');
% persistent ts;
% if isempty(ts)
%     ts=0;
%     %m_mem=zeros(10*1000,1);
% end
%m_mem(1:end-1)=m_mem(2:end);
%m_mem(end)=m(1);

%scale extension
% if(m(1)>0)
    a_pw=a_pw./pw_trace_max;%normalise of thw pw value chose to correspond to 1.
% elseif m(1)<0
%     m(1)=m(1)/max_flex;
% end
    
%ts=ts+1;
 trap1=trap;
 
 fdk=a_pw(1)-a_pw(2);%in this way the direction and magnitude of fdk tels which feedback is bigger(+ve for ED and -ve for FDS)
 
%stopSingnal=0;
%  if(ts==length(trap))
%      stopSingnal=1;
%  end

== matlab function EMG_FES2(backup-18-05-2018)/Voluntary +passive movement/Motor to FES/Tracing/TraceFcn_lowrate ==
  settings: sampleTime=1/50
  data: trap input; fbk input; trap1 output; fbk1 output
function  [trap1,fbk1]=fcn(trap,fbk)
%#codegen
% External MATLAB function connects to this block to read the values of the
% inputs. The external function is called whenever this block executes. So
% run this bloch at a low rate to reduce the rate of the external function
% which may be doing heavy activities like graphics



trap1=trap;
fbk1=fbk;

== matlab function EMG_FES2(backup-18-05-2018)/Voluntary +passive movement/Preprocessing/Signal conversion ==
  data: u input; y output; emgFR input
function y = fcn(u,emgFR)
%#codegen
%
% We will convert all signal to millivots athough the goniometer should be
% converted to degrees; we will just convert it to some randomly chosen
% range for now. B/C of the implementation in the reference block the
% randomly chosen range should be [-2,2].  WE WILL COME BACK HERE TO
% CONVERT TO ANGLE INSTEAD WHEN THE IMPLEMENTATION IN THE REFERENCE BLOCK
% CHANGES TO ANGLES
y=u;

% First convert Gonio
x=[-2,2]; %Range based on the Reference block/sub system
y(1) = (x(2)-x(1))*((u(1)-0)/(4-0))+x(1);% The analogue input still ranges from 0-4V

% Now for EMG
x=emgFR;
y(2:3)=(x(2)-x(1))*((u(2:3)-0)/(4-0))+x(1);%The analogue input still ranges from 0-4V
